simulink library "SimulinkToXPlane11"  (R2023a)
settings: Solver=VariableStepAuto  StartTime=0.0  StopTime=10.0  RelTol=1e-3
undefined symbols (not defined in the file or in its folder): SendPositionOrientationToXPlaneOverUDP
libraries: svdutilitieslib x1, dspnetwork x1
settings Model: Creator=LSV-PC0  LastModifiedBy=LSV-PC0

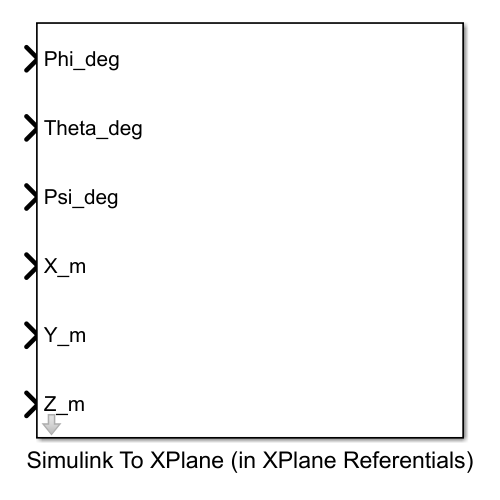
[thumbnail: Simulink's stored preview of the top-level diagram]
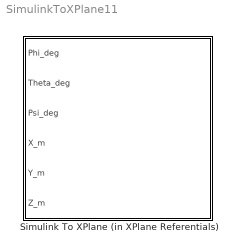
== system SimulinkToXPlane11 ==
  Simulink To XPlane (in XPlane Referentials) : Subsystem  mask{Precision=5}
      mask prompts: Precision "Insert here the precision"

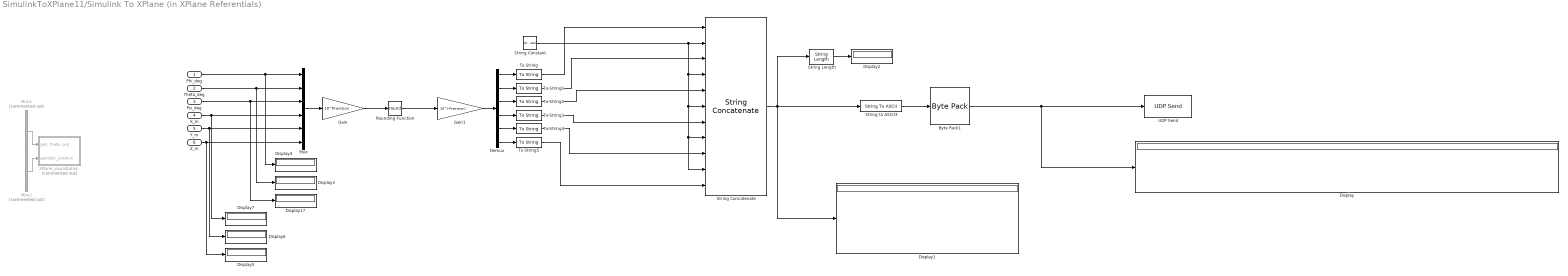
== system SimulinkToXPlane11/Simulink To XPlane (in XPlane Referentials) ==
  Phi_deg : Inport  PortDimensions=[1]
  Theta_deg : Inport  Port=2  PortDimensions=[1]
  Psi_deg : Inport  Port=3  PortDimensions=[1]
  X_m : Inport  Port=4  PortDimensions=[1]
  Y_m : Inport  Port=5  PortDimensions=[1]
  Z_m : Inport  Port=6  PortDimensions=[1]
  Byte Pack1 : svdutilitieslib/Byte Pack  maskPackedDataType=uint8  datatypes={'uint8'}  byteAlign=1  blockPlatform=arduinoert
  Demux : Demux  Outputs=6
  Display{,1..7,17} (9 alike) : Display
  Gain : Gain  Gain=10^Precision
  Gain1 : Gain  Gain=10^(-Precision)
  Mux : Mux  Inputs=6
  Mux1 : Mux  Commented=on  Inputs=3
  Mux2 : Mux  Commented=on  Inputs=3
  Rounding Function : Rounding  Operator=round
  String Concatenate : StringConcatenate  Inputs=11
  String Constant : StringConstant  String="\" \""
  String Length : StringLength
  String to ASCII3 : StringToASCII  OutputVectorSize=64
  To String{,1..5} (6 alike) : ToString
  UDP Send : dspnetwork/UDP Send  remoteURL='127.0.0.1'  remotePort=49003  localURL='0.0.0.0'  localPortSource=Automatically determine  localPort=-1  sendBufferSize=512  sampletime=-1  blockPlatform=[]  separateLengthPort=0
  XPlane_visualization : Subsystem  Commented=on  mask{IP_address='127.0.0.1', plugin_listening_port_number=49003, numDigitsOfPrecision=5}
      mask prompts: IP_address "String of X-Plane machine IP address (i.e. '192.168..112')"; plugin_listening_port_number "Port number that the X-Plane plugin is expecting to receive UDP messages on (i.e. 49003)"; numDigitsOfPrecision "Number of degrees of precision to transmit a string representation of a number over UDP (i.e. 10)"
      mask help:
      | Visualize state of aircraft using X-Plane.
      |
      | The machine running X-Plane should have a plugin operating which disables the internal X-Plane physics engine and listens to state information over UDP (which it then applies to the simulator).
      |
      | INPUT:
      | -3-by-1 vector of the euler angles [phi (rad);theta (rad);psi (rad)]
      | -geodetic_position: 3-by-1 vector of [latitude (rad); longitude (rad); altitude (m)]
      |
      | OUTPUT: -none
      |
      | Christopher Lum
      | lum@uw.edu
  wires:
  Byte Pack1/1 -> UDP Send/1, Display/1
  String to ASCII3/1 -> Byte Pack1/1
  To String/1 -> String Concatenate/1
  Demux/1 -> To String/1
  Demux/2 -> To String1/1
  To String1/1 -> String Concatenate/3
  To String2/1 -> String Concatenate/5
  Demux/3 -> To String2/1
  Demux/4 -> To String3/1
  Demux/5 -> To String4/1
  Gain/1 -> Rounding Function/1
  Rounding Function/1 -> Gain1/1
  Gain1/1 -> Demux/1
  Demux/6 -> To String5/1
  Mux/1 -> Gain/1
  String Concatenate/1 -> Display1/1, String Length/1, String to ASCII3/1
  String Constant/1 -> String Concatenate/10, String Concatenate/8, String Concatenate/6, String Concatenate/4, String Concatenate/2
  To String3/1 -> String Concatenate/7
  To String5/1 -> String Concatenate/11
  To String4/1 -> String Concatenate/9
  String Length/1 -> Display2/1
  Mux1/1 -> XPlane_visualization/1("[phi, theta, psi]")
  Mux2/1 -> XPlane_visualization/2(geodetic_position)
  X_m/1 -> Display7/1, Mux/4
  Psi_deg/1 -> Display17/1, Mux/3
  Theta_deg/1 -> Display3/1, Mux/2
  Phi_deg/1 -> Display4/1, Mux/1
  Z_m/1 -> Display5/1, Mux/6
  Y_m/1 -> Display6/1, Mux/5

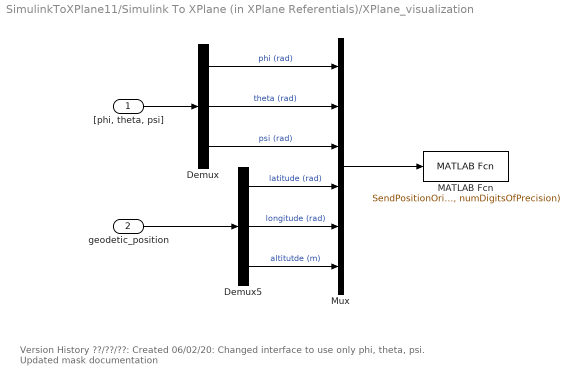
== system SimulinkToXPlane11/Simulink To XPlane (in XPlane Referentials)/XPlane_visualization ==
  note: Version History
      | ??/??/??: Created
      | 06/02/20: Changed interface to use only phi, theta, psi.  Updated mask documentation
  "[phi, theta, psi]" : Inport
  geodetic_position : Inport  Port=2
  Demux : Demux  Outputs=3
  Demux5 : Demux  Outputs=3
  MATLAB Fcn : MATLABFcn  MATLABFcn=SendPositionOrientationToXPlaneOverUDP(u, IP_address, plugin_listening_port_number, numDigitsOfPrecision)  OutputDimensions=0
  Mux : Mux  Inputs=6
  wires:
  Demux5/3 -> Mux/6  "altitutde (m)"
  Demux5/2 -> Mux/5  "longitude (rad)"
  Demux5/1 -> Mux/4  "latitude (rad)"
  Demux/3 -> Mux/3  "psi (rad)"
  Demux/2 -> Mux/2  "theta (rad)"
  Demux/1 -> Mux/1  "phi (rad)"
  "[phi, theta, psi]"/1 -> Demux/1
  geodetic_position/1 -> Demux5/1
  Mux/1 -> MATLAB Fcn/1
